simulink model "v3"  (R2023a)
settings: Solver=VariableStepAuto  StartTime=0.0  StopTime=4  RelTol=1e-3
libraries: dspvision x9, simulink x7, commsrccod2 x6, dspsigops x4, dspfdesign x4, commfilt2 x3, commchan3 x1, commsink2 x1
settings Model: Creator=zizim  LastModifiedBy=zizim
settings OptimizationCC: BlockReduction=off  ConditionallyExecuteInputs=off

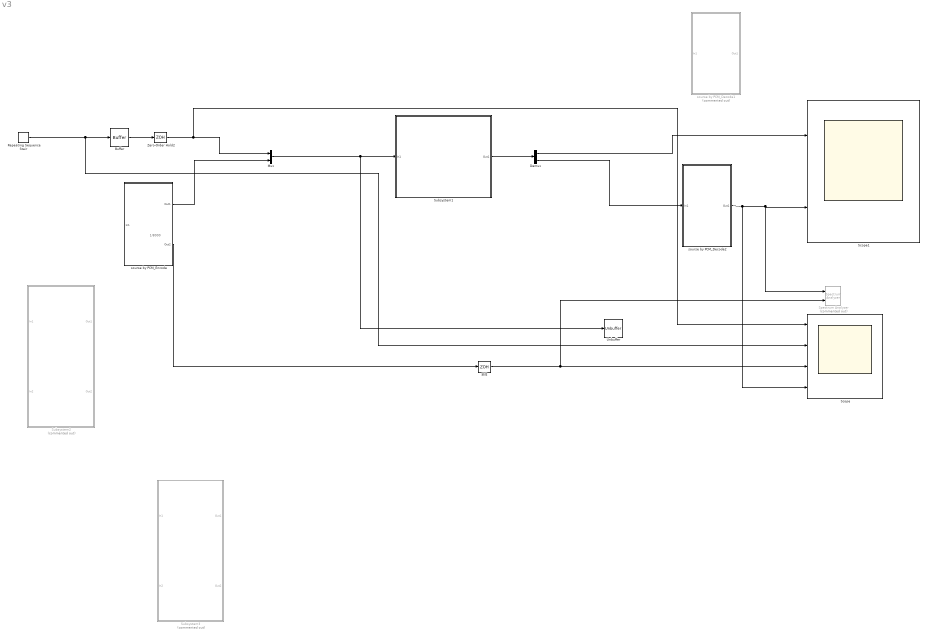
== system v3 ==
  note: 1/8000
  Buffer : Buffer  N=8  OutputFrames=off
  Demux : Demux  Outputs=2
  Mux : Mux  Inputs=2
  Repeating Sequence Stair : simulink/Sources/Repeating Sequence Stair  OutValues=[1 1 0 0 0 1 1 1]  tsamp=1/8000  OutMin=[]  OutMax=[]  OutDataTypeStr=double  OutputDataTypeScalingMode=double  OutDataType=fixdt(0,8)  ConRadixGroup=Best Precision: Vector-wise  OutScaling=2^-12
  Scope : Scope  NumInputPorts=4
  Scope1 : Scope  NumInputPorts=2
  Spectrum Analyzer : SpectrumAnalyzer  Commented=on  NumInputPorts=2  WindowPosition=[323.000000,237.000000,718.000000,504.000000,]  ScopeFrameLocation=window  Span=8000  StartFrequency=-4000  StopFrequency=4000  YLimits=[-105.37237061,9.4990938]  ColorLimits=[-80 20]  ShowLegend=on
  Subsystem1 : Subsystem
  Subsystem2 : Subsystem  Commented=on
  Subsystem3 : Subsystem  Commented=on
  Unbuffer : Unbuffer
  Zero-Order Hold2 : ZeroOrderHold  SampleTime=1/8000
  sourse by PCM_Decode1 : Subsystem  Commented=on
  sourse by PCM_Decode2 : Subsystem
  sourse by PCM_Encode : Subsystem
  采样 : ZeroOrderHold  SampleTime=1/64000
  wires:
  sourse by PCM_Encode/2(Out2) -> 采样/1
  采样/1 -> Spectrum Analyzer/2, Scope/3
  Mux/1 -> Unbuffer/1, Subsystem1/1(In1)
  sourse by PCM_Decode2/1(Out1) -> Scope/4, Spectrum Analyzer/1, Scope1/2
  Repeating Sequence Stair/1 -> Scope/2, Buffer/1
  Buffer/1 -> Zero-Order Hold2/1
  Zero-Order Hold2/1 -> Scope/1, Mux/1
  sourse by PCM_Encode/1(Out1) -> Mux/2
  Subsystem1/1(Out1) -> Demux/1
  Demux/2 -> sourse by PCM_Decode2/1(In1)
  Demux/1 -> Scope1/1

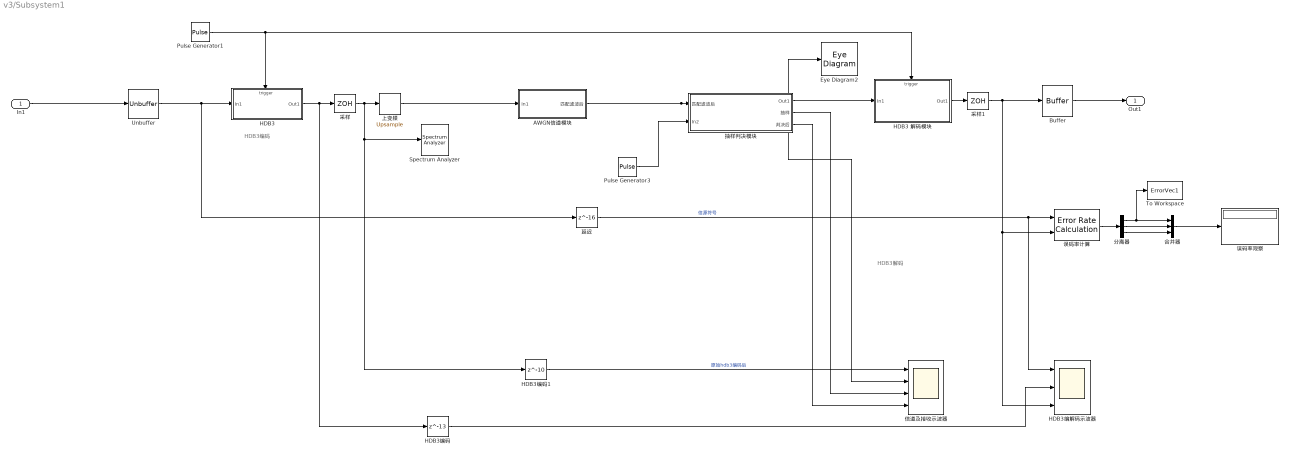
== system v3/Subsystem1 ==
  note: HDB3解码
  note: HDB3编码
  In1 : Inport
  AWGN信道模块 : Subsystem
  Buffer : Buffer  N=16  OutputFrames=off
  Eye Diagram2 : EyeDiagram
  HDB3 : Subsystem  TreatAsAtomicUnit=on
  HDB3 解码模块 : Subsystem  Tag=decode  Description=decode1  TreatAsAtomicUnit=on
  HDB3编码 : Delay  DelayLength=13  InitialCondition=0  SampleTime=1/128000
  HDB3编码1 : Delay  DelayLength=10  InitialCondition=0  SampleTime=1/128000
  HDB3编解码示波器 : Scope  NumInputPorts=3
  Pulse Generator1 : DiscretePulseGenerator  Period=10  PulseWidth=5  SampleTime=1/1280000
  Pulse Generator3 : DiscretePulseGenerator  Period=10  PulseWidth=5  SampleTime=1/1280000
  Spectrum Analyzer : SpectrumAnalyzer  WindowPosition=[507.000000,152.000000,800.000000,451.000000,]  ScopeFrameLocation=window  Method=Welch  SampleRate=1000  AxesScaling=Manual  Span=1000  StartFrequency=-500  StopFrequency=500  AveragingMethod=Running  YLimits=[-78.858739814638965981,15.222011316412805471]
      settings: OpenAtSimulationStart=off
  To Workspace : ToWorkspace  VariableName=ErrorVec1  SampleTime=-1
      settings: Save2DSignal=2-D array (concatenate along first dimension)
  Unbuffer : Unbuffer
  上变频 : dspsigops/Upsample  FactorSource=Dialog parameter  N=10  Nmax=16  phase=0  InputProcessing=Columns as channels (frame based)  RateOptions=Allow multirate processing  ic=0  mode=Unused parameter value
  信道及接收示波器 : Scope  NumInputPorts=4
  分离器 : Demux  Outputs=3
  合并器 : Mux  Inputs=3
  延迟 : Delay  DelayLength=16  InitialCondition=0  SampleTime=1/128000
  抽样判决模块 : Subsystem
  误码率观察 : Display
  误码率计算 : commsink2/Error Rate Calculation  N=0  st_delay=0  cp_mode=Entire frame  subframe=[]  PMode=Port  WsName=ErrorVec  RsMode2=off  stop=off  numErr=100  maxBits=1e6
  采样 : ZeroOrderHold  SampleTime=1/128000
  采样1 : ZeroOrderHold  SampleTime=1/128000
  Out1 : Outport
  wires:
  HDB3 解码模块/1(Out1) -> 采样1/1
  AWGN信道模块/1(匹配滤波后) -> 信道及接收示波器/2, Eye Diagram2/1, 抽样判决模块/1(匹配滤波后)
  分离器/2 -> 合并器/2
  采样/1 -> HDB3编码1/1, Spectrum Analyzer/1, 上变频/1
  HDB3/1(Out1) -> HDB3编码/1, 采样/1
  Pulse Generator1/1 -> HDB3 解码模块/Trigger, HDB3/Trigger
  分离器/3 -> 合并器/3
  上变频/1 -> AWGN信道模块/1(In1)
  抽样判决模块/2(抽样) -> 信道及接收示波器/3
  延迟/1 -> HDB3编解码示波器/1, 误码率计算/1  "信源符号"
  分离器/1 -> To Workspace/1, 合并器/1
  HDB3编码1/1 -> 信道及接收示波器/1  "原始hdb3编码后"
  合并器/1 -> 误码率观察/1
  Pulse Generator3/1 -> 抽样判决模块/2(In2)
  误码率计算/1 -> 分离器/1
  抽样判决模块/3(判决后) -> 信道及接收示波器/4
  HDB3编码/1 -> HDB3编解码示波器/2
  抽样判决模块/1(Out1) -> HDB3 解码模块/1(In1)
  采样1/1 -> Buffer/1, 误码率计算/2, HDB3编解码示波器/3
  In1/1 -> Unbuffer/1
  Unbuffer/1 -> 延迟/1, HDB3/1(In1)
  Buffer/1 -> Out1/1

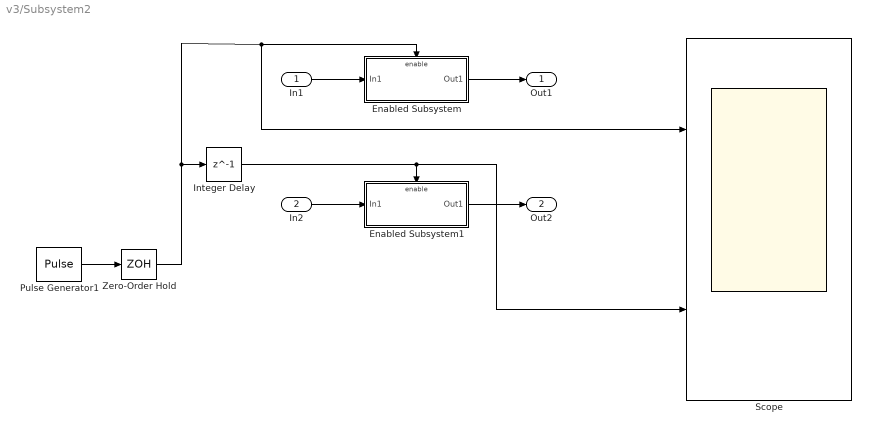
== system v3/Subsystem2 ==
  In1 : Inport
  In2 : Inport  Port=2
  Enabled Subsystem : Subsystem  TreatAsAtomicUnit=on
  Enabled Subsystem1 : Subsystem  TreatAsAtomicUnit=on
  Integer Delay : Delay  DelayLength=1
  Pulse Generator1 : DiscretePulseGenerator  PulseType=Time based  Amplitude=3  Period=1/160000  PulseWidth=1/320000  SampleTime=1/640000
  Scope : Scope  NumInputPorts=2
  Zero-Order Hold : ZeroOrderHold  SampleTime=1/320000
  Out1 : Outport
  Out2 : Outport  Port=2
  wires:
  Zero-Order Hold/1 -> Scope/1, Enabled Subsystem/Enable, Integer Delay/1
  Integer Delay/1 -> Scope/2, Enabled Subsystem1/Enable
  Pulse Generator1/1 -> Zero-Order Hold/1
  Enabled Subsystem/1(Out1) -> Out1/1
  In1/1 -> Enabled Subsystem/1(In1)
  In2/1 -> Enabled Subsystem1/1(In1)
  Enabled Subsystem1/1(Out1) -> Out2/1

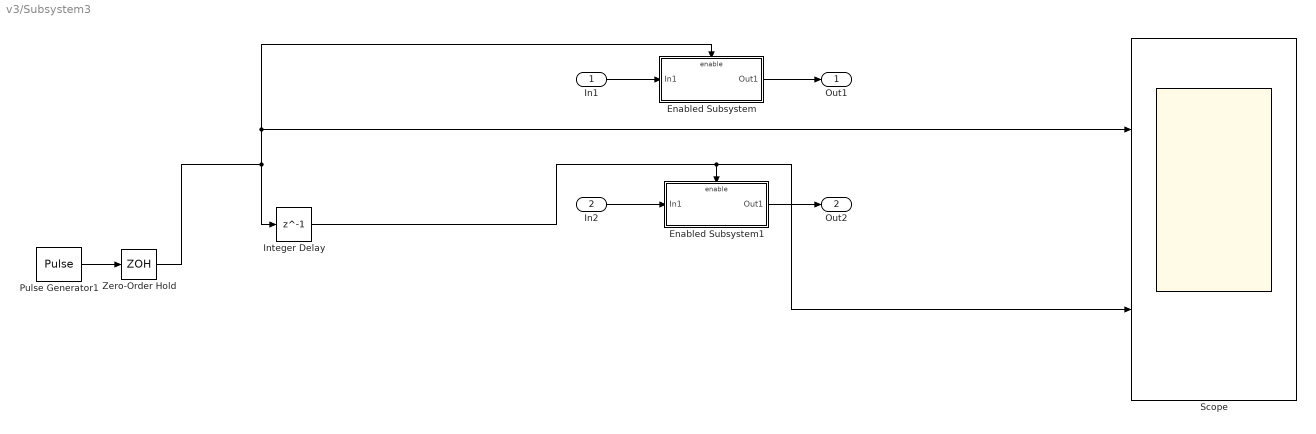
== system v3/Subsystem3 ==
  In1 : Inport
  In2 : Inport  Port=2
  Enabled Subsystem : Subsystem  TreatAsAtomicUnit=on
  Enabled Subsystem1 : Subsystem  TreatAsAtomicUnit=on
  Integer Delay : Delay  DelayLength=1
  Pulse Generator1 : DiscretePulseGenerator  PulseType=Time based  Amplitude=3  Period=1/160000  PulseWidth=1/320000  SampleTime=1/640000
  Scope : Scope  NumInputPorts=2
  Zero-Order Hold : ZeroOrderHold  SampleTime=1/32000
  Out1 : Outport
  Out2 : Outport  Port=2
  wires:
  Zero-Order Hold/1 -> Enabled Subsystem/Enable, Scope/1, Integer Delay/1
  Pulse Generator1/1 -> Zero-Order Hold/1
  Enabled Subsystem/1(Out1) -> Out1/1
  In1/1 -> Enabled Subsystem/1(In1)
  In2/1 -> Enabled Subsystem1/1(In1)
  Enabled Subsystem1/1(Out1) -> Out2/1
  Integer Delay/1 -> Scope/2, Enabled Subsystem1/Enable

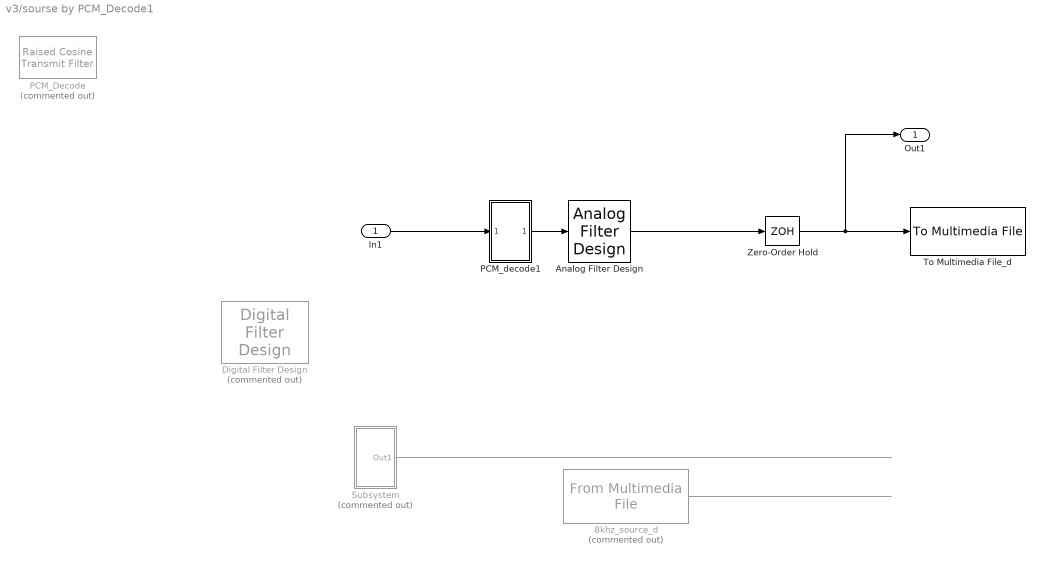
== system v3/sourse by PCM_Decode1 ==
  In1 : Inport
  8khz_source_d : dspvision/From Multimedia File  Commented=on  inputFilename=E:\Matlab\toolbox\dsp\samples\speech_dft_8kHz.wav  readRange=[1 Inf]  loop=on  numPlays=inf  outputStreams=Audio only  videoDataType=single  audioDataType=double  inheritSampleTime=on  userDefinedSampleTime=1/30  noAudioOutput=off  isIntensityVideo=off  fourcc=RGB  colorVideoFormat=Separate color signals  outputEOF=off  dataOrg=Column-major  audioFrameSize=1  computeAudioFrameSize=off  outSamplingMode=Sample based
      settings: LibrarySourceBlock=audiosources/From Multimedia File
  Analog Filter Design : dspfdesign/Analog Filter Design  method=Chebyshev II  filttype=Lowpass  N=8  Wlo=2*pi*3400  Whi=80  Rp=2  Rs=40
  Digital Filter Design : dspfdesign/Digital Filter Design  Commented=on  mwdsp_browser_bugfix_var=off
  PCM_Decode : commfilt2/Raised Cosine Transmit Filter  Commented=on  filtType=Square root  R=0.  filtSpan=10  N=8  filterGain=1  RateOptions=Allow multirate processing  framing=Mute  checkCoeff=off  variableName=rcTxFilt1  checkGain=Normalized  sampMode=Mute  saveAsFlag=0  currentFiltSpan=10  D=5  launchFVT=on  roundingMode=Floor  overflowMode=off  coeffDataTypeStr=Inherit: Same word length as input  coeffMin=[]  coeffMax=[]  coeffLastDataTypeStr=Inherit: Same word length as input  outputMin=[]  outputMax=[]
      settings: LibrarySourceBlock=|
      | commhdlfilt/Raised Cosine
      | Transmit Filter
  PCM_decode1 : Subsystem
  Subsystem : Subsystem  Commented=on
  To Multimedia File_d : dspvision/To Multimedia File  outputFilename=G:\zizim\Documents\code\Matlab\combine_system_hdb3\PCM_Decode_d.wav  streamSelection=Audio only  videoCompressor=None (uncompressed)  audioCompressor=None (uncompressed)  imagePorts=Separate color signals  fileType=WAV  audioDatatype=16-bit integer  fourcc=RGB  videoQuality=75  mj2000CompFactor=10
      settings: LibrarySourceBlock=audiosinks/To Multimedia File
  Zero-Order Hold : ZeroOrderHold  SampleTime=1/8000
  Out1 : Outport
  wires:
  Zero-Order Hold/1 -> Out1/1, To Multimedia File_d/1
  8khz_source_d/1 -> ?
  In1/1 -> PCM_decode1/1(In1)
  PCM_decode1/1(Out1) -> Analog Filter Design/1
  Subsystem/1(Out1) -> ?
  Analog Filter Design/1 -> Zero-Order Hold/1

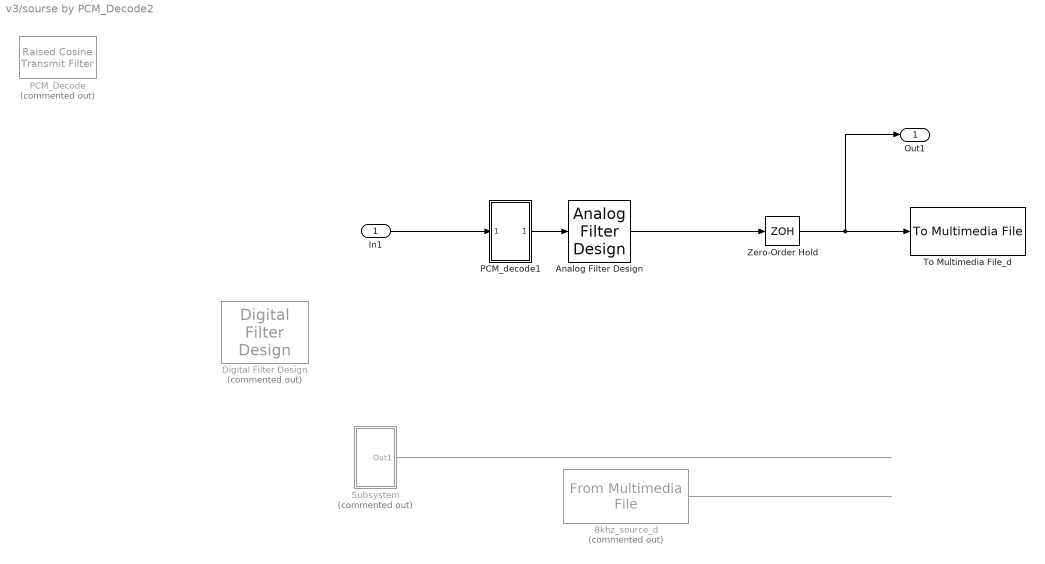
== system v3/sourse by PCM_Decode2 ==
  In1 : Inport
  8khz_source_d : dspvision/From Multimedia File  Commented=on  inputFilename=E:\Matlab\toolbox\dsp\samples\speech_dft_8kHz.wav  readRange=[1 Inf]  loop=on  numPlays=inf  outputStreams=Audio only  videoDataType=single  audioDataType=double  inheritSampleTime=on  userDefinedSampleTime=1/30  noAudioOutput=off  isIntensityVideo=off  fourcc=RGB  colorVideoFormat=Separate color signals  outputEOF=off  dataOrg=Column-major  audioFrameSize=1  computeAudioFrameSize=off  outSamplingMode=Sample based
      settings: LibrarySourceBlock=audiosources/From Multimedia File
  Analog Filter Design : dspfdesign/Analog Filter Design  method=Chebyshev II  filttype=Lowpass  N=8  Wlo=2*pi*3400  Whi=80  Rp=2  Rs=40
  Digital Filter Design : dspfdesign/Digital Filter Design  Commented=on  mwdsp_browser_bugfix_var=off
  PCM_Decode : commfilt2/Raised Cosine Transmit Filter  Commented=on  filtType=Square root  R=0.  filtSpan=10  N=8  filterGain=1  RateOptions=Allow multirate processing  framing=Mute  checkCoeff=off  variableName=rcTxFilt1  checkGain=Normalized  sampMode=Mute  saveAsFlag=0  currentFiltSpan=10  D=5  launchFVT=on  roundingMode=Floor  overflowMode=off  coeffDataTypeStr=Inherit: Same word length as input  coeffMin=[]  coeffMax=[]  coeffLastDataTypeStr=Inherit: Same word length as input  outputMin=[]  outputMax=[]
      settings: LibrarySourceBlock=|
      | commhdlfilt/Raised Cosine
      | Transmit Filter
  PCM_decode1 : Subsystem
  Subsystem : Subsystem  Commented=on
  To Multimedia File_d : dspvision/To Multimedia File  outputFilename=G:\zizim\Documents\UJN_HomeWork\通信原理仿真\communication_project\temp\PCM_Decode_d.wav  streamSelection=Audio only  videoCompressor=None (uncompressed)  audioCompressor=None (uncompressed)  imagePorts=Separate color signals  fileType=WAV  audioDatatype=16-bit integer  fourcc=RGB  videoQuality=75  mj2000CompFactor=10
      settings: LibrarySourceBlock=audiosinks/To Multimedia File
  Zero-Order Hold : ZeroOrderHold  SampleTime=1/8000
  Out1 : Outport
  wires:
  Zero-Order Hold/1 -> Out1/1, To Multimedia File_d/1
  8khz_source_d/1 -> ?
  In1/1 -> PCM_decode1/1(In1)
  PCM_decode1/1(Out1) -> Analog Filter Design/1
  Subsystem/1(Out1) -> ?
  Analog Filter Design/1 -> Zero-Order Hold/1

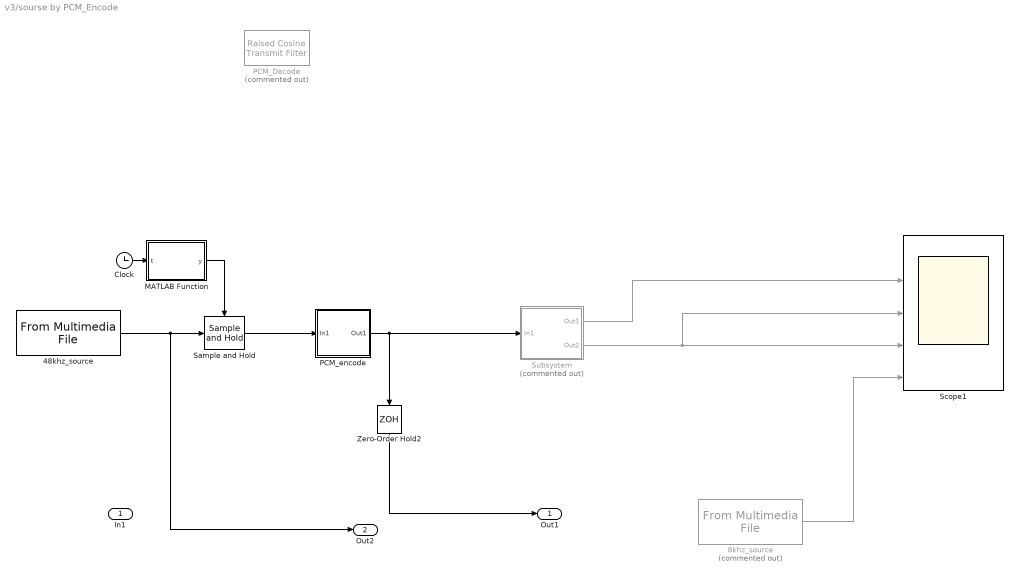
== system v3/sourse by PCM_Encode ==
  In1 : Inport
  48khz_source : dspvision/From Multimedia File  inputFilename=E:\Matlab\toolbox\dsp\samples\speech_dft_8kHz.wav  readRange=[1 Inf]  loop=on  numPlays=inf  outputStreams=Audio only  videoDataType=single  audioDataType=double  inheritSampleTime=on  userDefinedSampleTime=1/30  noAudioOutput=off  isIntensityVideo=off  fourcc=RGB  colorVideoFormat=Separate color signals  outputEOF=off  dataOrg=Column-major  audioFrameSize=1  computeAudioFrameSize=off  outSamplingMode=Sample based
      settings: LibrarySourceBlock=audiosources/From Multimedia File
  8khz_source : dspvision/From Multimedia File  Commented=on  inputFilename=E:\Matlab\toolbox\dsp\samples\speech_dft_8kHz.wav  readRange=[1 Inf]  loop=on  numPlays=inf  outputStreams=Audio only  videoDataType=single  audioDataType=double  inheritSampleTime=on  userDefinedSampleTime=1/30  noAudioOutput=off  isIntensityVideo=off  fourcc=RGB  colorVideoFormat=Separate color signals  outputEOF=off  dataOrg=Column-major  audioFrameSize=1  computeAudioFrameSize=off  outSamplingMode=Sample based
      settings: LibrarySourceBlock=audiosources/From Multimedia File
  Clock : Clock
      settings: Decimation=4
  MATLAB Function : MATLAB Function  TreatAsAtomicUnit=on
  PCM_Decode : commfilt2/Raised Cosine Transmit Filter  Commented=on  filtType=Square root  R=0.  filtSpan=10  N=8  filterGain=1  RateOptions=Allow multirate processing  framing=Mute  checkCoeff=off  variableName=rcTxFilt1  checkGain=Normalized  sampMode=Mute  saveAsFlag=0  currentFiltSpan=10  D=5  launchFVT=on  roundingMode=Floor  overflowMode=off  coeffDataTypeStr=Inherit: Same word length as input  coeffMin=[]  coeffMax=[]  coeffLastDataTypeStr=Inherit: Same word length as input  outputMin=[]  outputMax=[]
      settings: LibrarySourceBlock=|
      | commhdlfilt/Raised Cosine
      | Transmit Filter
  PCM_encode : Subsystem
  Sample and Hold : dspsigops/Sample and Hold  trig=Rising edge  initCond=0  latchinput=off
  Scope1 : Scope  NumInputPorts=5
  Subsystem : Subsystem  Commented=on
  Zero-Order Hold2 : ZeroOrderHold  SampleTime=1/8000
  Out1 : Outport
  Out2 : Outport  Port=2
  wires:
  8khz_source/1 -> Scope1/5
  Clock/1 -> MATLAB Function/1(t)
  MATLAB Function/1(y) -> Sample and Hold/Trigger
  Sample and Hold/1 -> PCM_encode/1(In1)
  Subsystem/2(Out2) -> Scope1/3, Scope1/4
  Subsystem/1(Out1) -> Scope1/2
  48khz_source/1 -> Out2/1, Sample and Hold/1
  PCM_encode/1(Out1) -> Zero-Order Hold2/1, Subsystem/1(In1)
  Zero-Order Hold2/1 -> Out1/1

== system v3/Subsystem1/AWGN信道模块 ==
  note: 信道模块
  In1 : Inport
  信道 : commchan3/AWGN Channel  LegacyMode=on  NoiseMethod="Signal to noise ratio  (SNR)"  noiseMode="Signal to noise ratio  (SNR)"  EbNo=10  EsNo=10  SNR=10000  BitsPerSymbol=1  SignalPower=1  SamplesPerSymbol=1  SymbolPeriod=1  VarianceSource=Parameter  Variance=1  RandomStream=Global stream  Seed=67  SimulateUsing=Code generation
  匹配滤波器 : DiscreteFilter  Numerator=[ rcosdesign(0.2,10,10,'sqrt')]  Denominator=[1]  SampleTime=1/1280000
  发射滤波器 : DiscreteFilter  Numerator=[ rcosdesign(0.2,10,10,'sqrt')]  Denominator=[1]  SampleTime=1/1280000
  匹配滤波后 : Outport
  wires:
  匹配滤波器/1 -> 匹配滤波后/1  "匹配滤波后"
  信道/1 -> 匹配滤波器/1
  In1/1 -> 发射滤波器/1
  发射滤波器/1 -> 信道/1

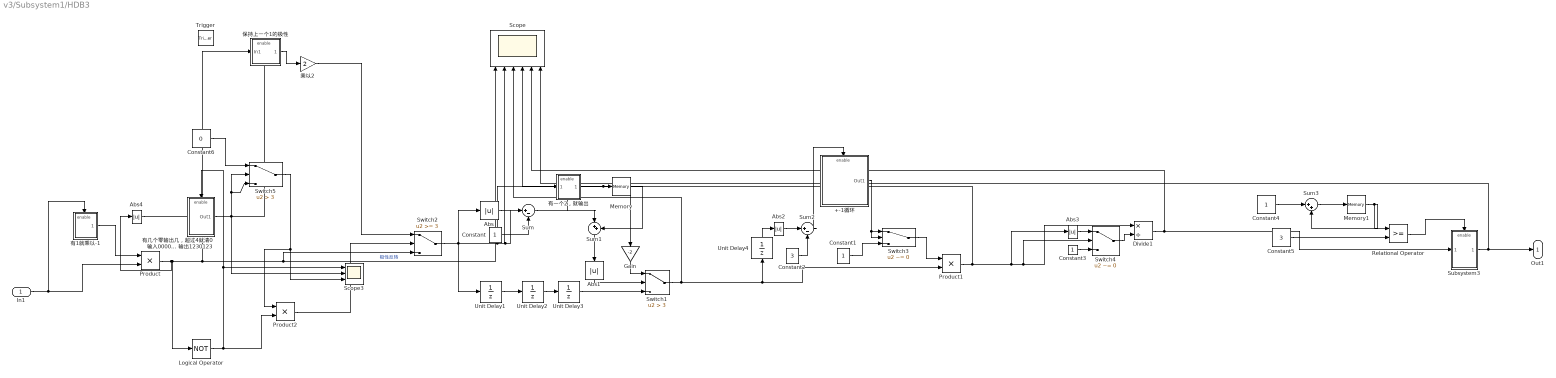
== system v3/Subsystem1/HDB3 ==
  In1 : Inport
  Trigger : TriggerPort  VariantControl=Variant
  +-1循环 : Subsystem
  Abs{,1..4} (5 alike) : Abs  SaturateOnIntegerOverflow=off
  Constant{,1,3..4} (4 alike) : Constant
  Constant2 : Constant  Value=3
  Constant5 : Constant  Value=3
  Constant6 : Constant  Value=0
  Divide1 : Product  Inputs=*/
  Gain : Gain  Gain=-2
  Logical Operator : Logic  Operator=NOT  AllPortsSameDT=off  OutDataTypeStr=boolean
  Memory : Memory  InheritSampleTime=on
  Memory1 : Memory  InheritSampleTime=on
  Product : Product  RndMeth=Zero
  Product1 : Product  RndMeth=Zero
  Product2 : Product  RndMeth=Zero
  Relational Operator : RelationalOperator  OutDataTypeStr=boolean  InputSameDT=off
  Scope : Scope  NumInputPorts=6
  Scope3 : Scope  NumInputPorts=3
  Subsystem3 : Subsystem
  Sum : Sum  Inputs=|+-
  Sum1 : Sum  Inputs=|++
  Sum2 : Sum  Inputs=|+-
  Sum3 : Sum  Inputs=|++
  Switch1 : Switch  Criteria=u2 > Threshold  Threshold=3  SaturateOnIntegerOverflow=off  InputSameDT=off
  Switch2 : Switch  Threshold=3  SaturateOnIntegerOverflow=off  InputSameDT=off
  Switch3 : Switch  Criteria=u2 ~= 0  Threshold=3  SaturateOnIntegerOverflow=off  InputSameDT=off
  Switch4 : Switch  Criteria=u2 ~= 0  Threshold=3  SaturateOnIntegerOverflow=off  InputSameDT=off
  Switch5 : Switch  Criteria=u2 > Threshold  Threshold=3  SaturateOnIntegerOverflow=off  InputSameDT=off
  Unit Delay{1..4} (4 alike) : UnitDelay  SampleTime=-1  HasFrameUpgradeWarning=on
  乘以2 : Gain  Gain=2
  保持上一个1的极性 : Subsystem
  有1就乘以-1 : Subsystem
  有一个2，就输出 : Subsystem
  有几个零输出几，超过4就清0 输入0000000 输出1230123 : Subsystem
  Out1 : Outport
  wires:
  In1/1 -> 有1就乘以-1/Enable, Product/2
  Memory1/1 -> Sum3/2, Relational Operator/1
  Subsystem3/1(Out1) -> Out1/1, Scope/6
  Constant5/1 -> Relational Operator/2
  Relational Operator/1 -> Subsystem3/Enable
  Divide1/1 -> Scope/5, Subsystem3/1(In2)
  Constant4/1 -> Sum3/1
  Sum3/1 -> Memory1/1
  Sum1/1 -> Abs1/1
  Abs1/1 -> Switch1/2
  Abs/1 -> Sum/1
  Sum2/1 -> +-1循环/Enable
  Constant/1 -> Sum/2
  Sum/1 -> 有一个2，就输出/Enable
  +-1循环/1(Out1) -> Switch3/2, Switch3/1
  有一个2，就输出/1(Out1) -> Gain/1, Memory/1
  Memory/1 -> Sum1/2
  Unit Delay3/1 -> Switch1/3
  Gain/1 -> Switch1/1
  Unit Delay1/1 -> Unit Delay2/1
  Switch3/1 -> Product1/1
  Switch4/1 -> Divide1/2
  Constant2/1 -> Sum2/2
  Switch1/1 -> Product1/2, Unit Delay4/1, Scope/3
  Unit Delay4/1 -> Abs2/1
  Abs3/1 -> Switch4/1
  Abs2/1 -> Sum2/1
  Constant3/1 -> Switch4/3
  Constant1/1 -> Switch3/3
  乘以2/1 -> Switch2/1
  Product1/1 -> Switch4/2, Divide1/1, Abs3/1, Scope/4
  有1就乘以-1/1(Out1) -> Product/1
  Product/1 -> Switch2/3, Scope/1, 保持上一个1的极性/1(In1), Logical Operator/1, Abs4/1  "极性反转"
  Unit Delay2/1 -> Unit Delay3/1
  Switch2/1 -> Sum1/1, Scope/2, 有一个2，就输出/1(In1), Abs/1, Unit Delay1/1
  保持上一个1的极性/1(Out1) -> 乘以2/1
  Product2/1 -> Switch2/2
  Abs4/1 -> 保持上一个1的极性/Enable
  有几个零输出几，超过4就清0 输入0000000 输出1230123/1(Out1) -> Switch5/3, Switch5/2, Scope3/2
  Constant6/1 -> Switch5/1
  Logical Operator/1 -> Product2/2, 有几个零输出几，超过4就清0 输入0000000 输出1230123/Enable, Scope3/1
  Switch5/1 -> Product2/1, Scope3/3

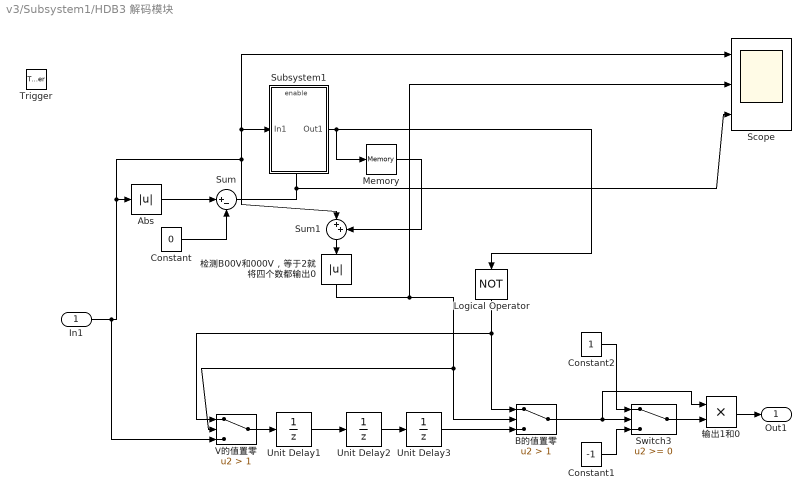
== system v3/Subsystem1/HDB3 解码模块 ==
  In1 : Inport
  Trigger : TriggerPort  VariantControl=Variant
  Abs : Abs  SaturateOnIntegerOverflow=off
  B的值置零 : Switch  Criteria=u2 > Threshold  Threshold=1  SaturateOnIntegerOverflow=off  InputSameDT=off
  Constant : Constant  Value=0
  Constant1 : Constant  Value=-1
  Constant2 : Constant
  Logical Operator : Logic  Operator=NOT  AllPortsSameDT=off  OutDataTypeStr=boolean
  Memory : Memory  InheritSampleTime=on
  Scope : Scope  NumInputPorts=3
  Subsystem1 : Subsystem
  Sum : Sum  Inputs=|+-
  Sum1 : Sum  Inputs=|++
  Switch3 : Switch  SaturateOnIntegerOverflow=off  InputSameDT=off
  Unit Delay1 : UnitDelay  SampleTime=-1  HasFrameUpgradeWarning=on
  Unit Delay2 : UnitDelay  SampleTime=-1  HasFrameUpgradeWarning=on
  Unit Delay3 : UnitDelay  SampleTime=-1  HasFrameUpgradeWarning=on
  V的值置零 : Switch  Criteria=u2 > Threshold  Threshold=1  SaturateOnIntegerOverflow=off  InputSameDT=off
  检测B00V和000V，等于2就将四个数都输出0 : Abs  SaturateOnIntegerOverflow=off
  输出1和0 : Product  RndMeth=Zero
  Out1 : Outport
  wires:
  In1/1 -> V的值置零/3, Subsystem1/1(In1), Scope/1, Sum1/1, Abs/1
  Constant/1 -> Sum/2
  Abs/1 -> Sum/1
  Sum/1 -> Scope/3, Subsystem1/Enable
  Subsystem1/1(Out1) -> Memory/1, Logical Operator/1
  Memory/1 -> Sum1/2
  Sum1/1 -> 检测B00V和000V，等于2就将四个数都输出0/1
  检测B00V和000V，等于2就将四个数都输出0/1 -> Scope/2, B的值置零/2, V的值置零/2
  Logical Operator/1 -> V的值置零/1, B的值置零/1
  Unit Delay3/1 -> B的值置零/3
  Unit Delay1/1 -> Unit Delay2/1
  Unit Delay2/1 -> Unit Delay3/1
  V的值置零/1 -> Unit Delay1/1
  B的值置零/1 -> Switch3/2, 输出1和0/1
  Constant1/1 -> Switch3/3
  Constant2/1 -> Switch3/1
  Switch3/1 -> 输出1和0/2
  输出1和0/1 -> Out1/1

== system v3/Subsystem1/抽样判决模块 ==
  匹配滤波后 : Inport
  In2 : Inport  Port=2
  Downsample1 : DownSample  N=10  InputProcessing=Inherited (this choice will be removed - see release notes)  RateOptions=Allow multirate processing
  判决 : Subsystem
  每隔抽样 : Subsystem  TreatAsAtomicUnit=on
  Out1 : Outport
  抽样 : Outport  Port=2
  判决后 : Outport  Port=3
  wires:
  Downsample1/1 -> Out1/1
  匹配滤波后/1 -> 每隔抽样/1(In1)
  判决/1(Out1) -> 判决后/1, Downsample1/1  "判决后"
  每隔抽样/1(Out1) -> 抽样/1, 判决/1(In1)  "抽样"
  In2/1 -> 每隔抽样/Trigger

== system v3/Subsystem2/Enabled Subsystem ==
  In1 : Inport
  Enable : EnablePort
  Out1 : Outport
  wires:
  In1/1 -> Out1/1

== system v3/Subsystem2/Enabled Subsystem1 ==
  In1 : Inport
  Enable : EnablePort
  Out1 : Outport
  wires:
  In1/1 -> Out1/1

== system v3/Subsystem3/Enabled Subsystem ==
  In1 : Inport
  Enable : EnablePort
  Out1 : Outport
  wires:
  In1/1 -> Out1/1

== system v3/Subsystem3/Enabled Subsystem1 ==
  In1 : Inport
  Enable : EnablePort
  Out1 : Outport
  wires:
  In1/1 -> Out1/1

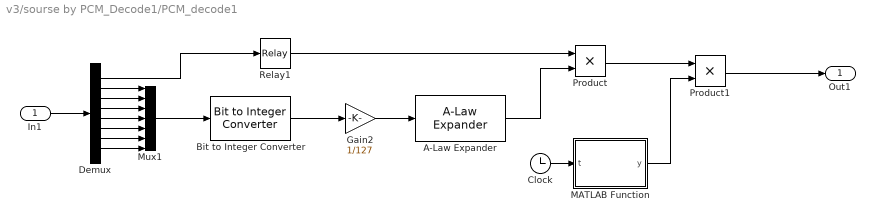
== system v3/sourse by PCM_Decode1/PCM_decode1 ==
  In1 : Inport
  A-Law Expander : commsrccod2/A-Law Expander  A=87.6  V=1
  Bit to Integer Converter : simulink/Logic and Bit Operations/Bit to Integer Converter  nbits=7  bitOrder=MSB first  signedOutputValues=Unsigned  outDtype=double  outDtypeSigned=Inherit via internal rule
      settings: LibrarySourceBlock=|
      | commutil2/Bit to Integer
      | Converter
  Clock : Clock
      settings: Decimation=4
  Demux : Demux  Outputs=8
  Gain2 : Gain  Gain=1/127
  MATLAB Function : MATLAB Function  TreatAsAtomicUnit=on
  Mux1 : Mux  Inputs=7
  Product : Product
  Product1 : Product
  Relay1 : Relay  OnSwitchValue=0.9  OffOutputValue=-1
  Out1 : Outport
  wires:
  In1/1 -> Demux/1
  Relay1/1 -> Product/1
  Demux/5 -> Mux1/4
  Mux1/1 -> Bit to Integer Converter/1
  Demux/1 -> Relay1/1
  Demux/4 -> Mux1/3
  Gain2/1 -> A-Law Expander/1
  Demux/6 -> Mux1/5
  Demux/7 -> Mux1/6
  Bit to Integer Converter/1 -> Gain2/1
  Demux/2 -> Mux1/1
  Demux/3 -> Mux1/2
  A-Law Expander/1 -> Product/2
  Demux/8 -> Mux1/7
  Product/1 -> Product1/1
  Product1/1 -> Out1/1
  MATLAB Function/1(y) -> Product1/2
  Clock/1 -> MATLAB Function/1(t)

== system v3/sourse by PCM_Decode1/Subsystem ==
  48khz_source_d : dspvision/From Multimedia File  inputFilename=E:\Matlab\toolbox\dsp\samples\audio48kHz.wav  readRange=[1 Inf]  loop=on  numPlays=inf  outputStreams=Audio only  videoDataType=single  audioDataType=double  inheritSampleTime=on  userDefinedSampleTime=1/30  noAudioOutput=off  isIntensityVideo=off  fourcc=RGB  colorVideoFormat=Separate color signals  outputEOF=off  dataOrg=Column-major  audioFrameSize=1  computeAudioFrameSize=off  outSamplingMode=Sample based
      settings: LibrarySourceBlock=audiosources/From Multimedia File
  Clock : Clock
      settings: Decimation=4
  MATLAB Function : MATLAB Function  TreatAsAtomicUnit=on
  PCM_encode_d : Subsystem
  Sample and Hold : dspsigops/Sample and Hold  trig=Rising edge  initCond=0  latchinput=off
  Out1 : Outport
  wires:
  Clock/1 -> MATLAB Function/1(t)
  Sample and Hold/1 -> PCM_encode_d/1(In1)
  48khz_source_d/1 -> Sample and Hold/1
  MATLAB Function/1(y) -> Sample and Hold/Trigger
  PCM_encode_d/1(Out1) -> Out1/1

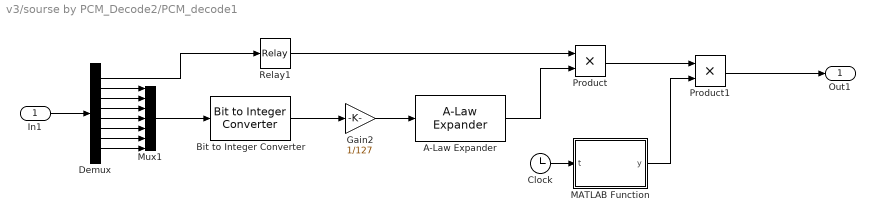
== system v3/sourse by PCM_Decode2/PCM_decode1 ==
  In1 : Inport
  A-Law Expander : commsrccod2/A-Law Expander  A=87.6  V=1
  Bit to Integer Converter : simulink/Logic and Bit Operations/Bit to Integer Converter  nbits=7  bitOrder=MSB first  signedOutputValues=Unsigned  outDtype=double  outDtypeSigned=Inherit via internal rule
      settings: LibrarySourceBlock=|
      | commutil2/Bit to Integer
      | Converter
  Clock : Clock
      settings: Decimation=4
  Demux : Demux  Outputs=8
  Gain2 : Gain  Gain=1/127
  MATLAB Function : MATLAB Function  TreatAsAtomicUnit=on
  Mux1 : Mux  Inputs=7
  Product : Product
  Product1 : Product
  Relay1 : Relay  OnSwitchValue=0.9  OffOutputValue=-1
  Out1 : Outport
  wires:
  In1/1 -> Demux/1
  Relay1/1 -> Product/1
  Demux/5 -> Mux1/4
  Mux1/1 -> Bit to Integer Converter/1
  Demux/1 -> Relay1/1
  Demux/4 -> Mux1/3
  Gain2/1 -> A-Law Expander/1
  Demux/6 -> Mux1/5
  Demux/7 -> Mux1/6
  Bit to Integer Converter/1 -> Gain2/1
  Demux/2 -> Mux1/1
  Demux/3 -> Mux1/2
  A-Law Expander/1 -> Product/2
  Demux/8 -> Mux1/7
  Product/1 -> Product1/1
  Product1/1 -> Out1/1
  MATLAB Function/1(y) -> Product1/2
  Clock/1 -> MATLAB Function/1(t)

== system v3/sourse by PCM_Decode2/Subsystem ==
  48khz_source_d : dspvision/From Multimedia File  inputFilename=E:\Matlab\toolbox\dsp\samples\audio48kHz.wav  readRange=[1 Inf]  loop=on  numPlays=inf  outputStreams=Audio only  videoDataType=single  audioDataType=double  inheritSampleTime=on  userDefinedSampleTime=1/30  noAudioOutput=off  isIntensityVideo=off  fourcc=RGB  colorVideoFormat=Separate color signals  outputEOF=off  dataOrg=Column-major  audioFrameSize=1  computeAudioFrameSize=off  outSamplingMode=Sample based
      settings: LibrarySourceBlock=audiosources/From Multimedia File
  Clock : Clock
      settings: Decimation=4
  MATLAB Function : MATLAB Function  TreatAsAtomicUnit=on
  PCM_encode_d : Subsystem
  Sample and Hold : dspsigops/Sample and Hold  trig=Rising edge  initCond=0  latchinput=off
  Out1 : Outport
  wires:
  Clock/1 -> MATLAB Function/1(t)
  Sample and Hold/1 -> PCM_encode_d/1(In1)
  48khz_source_d/1 -> Sample and Hold/1
  MATLAB Function/1(y) -> Sample and Hold/Trigger
  PCM_encode_d/1(Out1) -> Out1/1

== system v3/sourse by PCM_Encode/PCM_encode ==
  In1 : Inport
  A-Law Compressor : commsrccod2/A-Law Compressor  A=87.6  V=1
  Abs : Abs  SaturateOnIntegerOverflow=off
  Gain1 : Gain  Gain=127
  Integer to Bit Converter : simulink/Logic and Bit Operations/Integer to Bit Converter  nbits=7  signedInputValues=Unsigned  bitOrder=MSB first  outDtype=Inherit via internal rule
      settings: LibrarySourceBlock=|
      | commutil2/Integer to Bit
      | Converter
  Mux : Mux  Inputs=2
  Quantizer : Quantizer  QuantizationInterval=1
  Relay : Relay
  Saturation : Saturate  UpperLimit=1  LowerLimit=-1
  Out1 : Outport
  wires:
  Integer to Bit Converter/1 -> Mux/2
  Mux/1 -> Out1/1
  A-Law Compressor/1 -> Gain1/1
  Gain1/1 -> Quantizer/1
  Quantizer/1 -> Integer to Bit Converter/1
  Saturation/1 -> Abs/1
  Relay/1 -> Mux/1
  Abs/1 -> Relay/1, A-Law Compressor/1
  In1/1 -> Saturation/1

== system v3/sourse by PCM_Encode/Subsystem ==
  In1 : Inport
  PCM_decode1 : Subsystem
  To Multimedia File : dspvision/To Multimedia File  outputFilename=G:\zizim\Documents\作业\audio_output\PCM_Decode.wav  streamSelection=Audio only  videoCompressor=None (uncompressed)  audioCompressor=None (uncompressed)  imagePorts=Separate color signals  fileType=WAV  audioDatatype=Determine from input data type  fourcc=RGB  videoQuality=75  mj2000CompFactor=10
      settings: LibrarySourceBlock=audiosinks/To Multimedia File
  Zero-Order Hold : ZeroOrderHold  SampleTime=-1
  Out1 : Outport
  Out2 : Outport  Port=2
  wires:
  PCM_decode1/1(Out1) -> Out1/1, Zero-Order Hold/1
  In1/1 -> PCM_decode1/1(In1)
  Zero-Order Hold/1 -> Out2/1, To Multimedia File/1

== system v3/Subsystem1/HDB3/+-1循环 ==
  Enable : EnablePort
  Constant1 : Constant  Value=-1
  Memory : Memory  InitialCondition=1  InheritSampleTime=on
  Product : Product  RndMeth=Zero
  Out1 : Outport
  wires:
  Constant1/1 -> Product/1
  Memory/1 -> Product/2
  Product/1 -> Memory/1, Out1/1

== system v3/Subsystem1/HDB3/Subsystem3 ==
  In2 : Inport
  Enable : EnablePort
  Out1 : Outport
  wires:
  In2/1 -> Out1/1

== system v3/Subsystem1/HDB3/保持上一个1的极性 ==
  In1 : Inport
  Enable : EnablePort  StatesWhenEnabling=reset
  Out1 : Outport
  wires:
  In1/1 -> Out1/1

== system v3/Subsystem1/HDB3/有1就乘以-1 ==
  Enable : EnablePort
  Constant1 : Constant  Value=-1
  Memory : Memory  InitialCondition=-1  InheritSampleTime=on
  Product : Product  RndMeth=Zero
  Out1 : Outport
  wires:
  Constant1/1 -> Product/1
  Memory/1 -> Product/2
  Product/1 -> Memory/1, Out1/1

== system v3/Subsystem1/HDB3/有一个2，就输出 ==
  In1 : Inport
  Enable : EnablePort  StatesWhenEnabling=reset
  Out1 : Outport
  wires:
  In1/1 -> Out1/1

== system v3/Subsystem1/HDB3/有几个零输出几，超过4就清0 输入0000000 输出1230123 ==
  Enable : EnablePort  StatesWhenEnabling=reset
  Add : Sum
  Constant : Constant
  Constant1 : Constant  Value=0
  Switch3 : Switch  Criteria=u2 > Threshold  Threshold=3  SaturateOnIntegerOverflow=off  InputSameDT=off
  Unit Delay : UnitDelay  SampleTime=-1  HasFrameUpgradeWarning=on
  Out1 : Outport
  wires:
  Constant/1 -> Add/1
  Add/1 -> Unit Delay/1
  Unit Delay/1 -> Switch3/2, Switch3/3
  Constant1/1 -> Switch3/1
  Switch3/1 -> Add/2, Out1/1

== system v3/Subsystem1/HDB3 解码模块/Subsystem1 ==
  In1 : Inport
  Enable : EnablePort  StatesWhenEnabling=reset
  Out1 : Outport
  wires:
  In1/1 -> Out1/1

== system v3/Subsystem1/抽样判决模块/判决 ==
  In1 : Inport
  Constant12 : Constant
  Constant13 : Constant  Value=0
  Constant14 : Constant  Value=-1
  Constant15 : Constant  Value=0
  Gain5 : Gain  Gain=-1
  Sum4 : Sum  Inputs=|++
  开关电路6 : Switch  Criteria=u2 > Threshold  Threshold=0.5  SaturateOnIntegerOverflow=off  InputSameDT=off
  开关电路7 : Switch  Criteria=u2 > Threshold  Threshold=0.5  SaturateOnIntegerOverflow=off  InputSameDT=off
  Out1 : Outport
  wires:
  Sum4/1 -> Out1/1
  In1/1 -> Gain5/1, 开关电路6/2
  Constant14/1 -> 开关电路7/1
  Constant13/1 -> 开关电路6/3
  开关电路6/1 -> Sum4/1
  开关电路7/1 -> Sum4/2
  Constant15/1 -> 开关电路7/3
  Constant12/1 -> 开关电路6/1
  Gain5/1 -> 开关电路7/2

== system v3/Subsystem1/抽样判决模块/每隔抽样 ==
  In1 : Inport
  Trigger : TriggerPort  VariantControl=Variant
  Out1 : Outport
  wires:
  In1/1 -> Out1/1

== system v3/sourse by PCM_Decode1/Subsystem/PCM_encode_d ==
  In1 : Inport
  A-Law Compressor : commsrccod2/A-Law Compressor  A=87.6  V=1
  Abs : Abs  SaturateOnIntegerOverflow=off
  Gain1 : Gain  Gain=127
  Integer to Bit Converter : simulink/Logic and Bit Operations/Integer to Bit Converter  nbits=7  signedInputValues=Unsigned  bitOrder=MSB first  outDtype=Inherit via internal rule
      settings: LibrarySourceBlock=|
      | commutil2/Integer to Bit
      | Converter
  Mux : Mux  Inputs=2
  Quantizer : Quantizer  QuantizationInterval=1
  Relay : Relay
  Saturation : Saturate  UpperLimit=1  LowerLimit=-1
  Out1 : Outport
  wires:
  Integer to Bit Converter/1 -> Mux/2
  Mux/1 -> Out1/1
  A-Law Compressor/1 -> Gain1/1
  Gain1/1 -> Quantizer/1
  Quantizer/1 -> Integer to Bit Converter/1
  Saturation/1 -> Abs/1
  Relay/1 -> Mux/1
  Abs/1 -> Relay/1, A-Law Compressor/1
  In1/1 -> Saturation/1

== system v3/sourse by PCM_Decode2/Subsystem/PCM_encode_d ==
  In1 : Inport
  A-Law Compressor : commsrccod2/A-Law Compressor  A=87.6  V=1
  Abs : Abs  SaturateOnIntegerOverflow=off
  Gain1 : Gain  Gain=127
  Integer to Bit Converter : simulink/Logic and Bit Operations/Integer to Bit Converter  nbits=7  signedInputValues=Unsigned  bitOrder=MSB first  outDtype=Inherit via internal rule
      settings: LibrarySourceBlock=|
      | commutil2/Integer to Bit
      | Converter
  Mux : Mux  Inputs=2
  Quantizer : Quantizer  QuantizationInterval=1
  Relay : Relay
  Saturation : Saturate  UpperLimit=1  LowerLimit=-1
  Out1 : Outport
  wires:
  Integer to Bit Converter/1 -> Mux/2
  Mux/1 -> Out1/1
  A-Law Compressor/1 -> Gain1/1
  Gain1/1 -> Quantizer/1
  Quantizer/1 -> Integer to Bit Converter/1
  Saturation/1 -> Abs/1
  Relay/1 -> Mux/1
  Abs/1 -> Relay/1, A-Law Compressor/1
  In1/1 -> Saturation/1

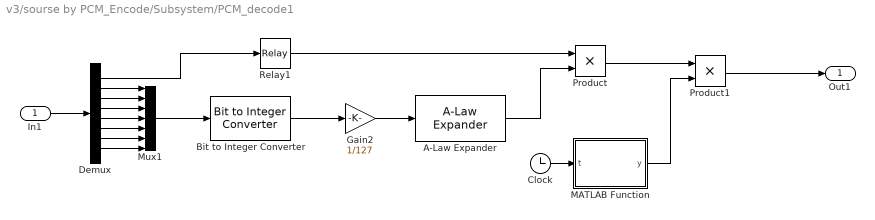
== system v3/sourse by PCM_Encode/Subsystem/PCM_decode1 ==
  In1 : Inport
  A-Law Expander : commsrccod2/A-Law Expander  A=87.6  V=1
  Bit to Integer Converter : simulink/Logic and Bit Operations/Bit to Integer Converter  nbits=7  bitOrder=MSB first  signedOutputValues=Unsigned  outDtype=double  outDtypeSigned=Inherit via internal rule
      settings: LibrarySourceBlock=|
      | commutil2/Bit to Integer
      | Converter
  Clock : Clock
      settings: Decimation=4
  Demux : Demux  Outputs=8
  Gain2 : Gain  Gain=1/127
  MATLAB Function : MATLAB Function  TreatAsAtomicUnit=on
  Mux1 : Mux  Inputs=7
  Product : Product
  Product1 : Product
  Relay1 : Relay  OnSwitchValue=0.9  OffOutputValue=-1
  Out1 : Outport
  wires:
  In1/1 -> Demux/1
  Relay1/1 -> Product/1
  Demux/5 -> Mux1/4
  Mux1/1 -> Bit to Integer Converter/1
  Demux/1 -> Relay1/1
  Demux/4 -> Mux1/3
  Gain2/1 -> A-Law Expander/1
  Demux/6 -> Mux1/5
  Demux/7 -> Mux1/6
  Bit to Integer Converter/1 -> Gain2/1
  Demux/2 -> Mux1/1
  Demux/3 -> Mux1/2
  A-Law Expander/1 -> Product/2
  Demux/8 -> Mux1/7
  Product/1 -> Product1/1
  Product1/1 -> Out1/1
  MATLAB Function/1(y) -> Product1/2
  Clock/1 -> MATLAB Function/1(t)

== matlab function v3/sourse by PCM_Encode/Subsystem/PCM_decode1/MATLAB Function ==
  data: t input; y output
function y = rect_wave(t)
    % 生成周期为1/(4*pi)、占空比50%、幅度在-1和1之间的矩形波
    % 输入t：Simulink仿真时间（需将模块输入连接到Clock模块的输出）
    
    T = 1/8000;  % 周期
    duty = 0.5;    % 占空比50%
    
    % 计算归一化时间（在0到周期内的位置）
    t_norm = mod(t, T);
    
    % 生成矩形波：前半周期为1，后半周期为-1
    if t_norm < duty * T
        y = 1;
    else
        y = -1;
    end
end

== matlab function v3/sourse by PCM_Decode1/PCM_decode1/MATLAB Function ==
  data: t input; y output
function y = rect_wave(t)
    % 生成周期为1/(4*pi)、占空比50%、幅度在-1和1之间的矩形波
    % 输入t：Simulink仿真时间（需将模块输入连接到Clock模块的输出）
    
    T = 1/8000;  % 周期
    duty = 0.5;    % 占空比50%
    
    % 计算归一化时间（在0到周期内的位置）
    t_norm = mod(t, T);
    
    % 生成矩形波：前半周期为1，后半周期为-1
    if t_norm < duty * T
        y = 1;
    else
        y = -1;
    end
end

== matlab function v3/sourse by PCM_Decode1/Subsystem/MATLAB Function ==
  data: t input; y output
function y = rect_wave(t)
    % 生成周期为1/(4*pi)、占空比50%、幅度在-1和1之间的矩形波
    % 输入t：Simulink仿真时间（需将模块输入连接到Clock模块的输出）
    
    T = 1/8000;  % 周期
    duty = 0.5;    % 占空比50%
    
    % 计算归一化时间（在0到周期内的位置）
    t_norm = mod(t, T);
    
    % 生成矩形波：前半周期为1，后半周期为-1
    if t_norm < duty * T
        y = 1;
    else
        y = -1;
    end
end

== matlab function v3/sourse by PCM_Encode/MATLAB Function ==
  data: t input; y output
function y = rect_wave(t)
    % 生成、占空比50%、幅度在-1和1之间的矩形波
    % 输入t：Simulink仿真时间（需将模块输入连接到Clock模块的输出）
    
    T = 1/8000;  % 周期
    duty = 0.5;    % 占空比50%
    
    % 计算归一化时间（在0到周期内的位置）
    t_norm = mod(t, T);
    
    % 生成矩形波：前半周期为1，后半周期为-1
    if t_norm < duty * T
        y = 1;
    else
        y = -1;
    end
end

== matlab function v3/sourse by PCM_Decode2/Subsystem/MATLAB Function ==
  data: t input; y output
function y = rect_wave(t)
    % 生成周期为1/(4*pi)、占空比50%、幅度在-1和1之间的矩形波
    % 输入t：Simulink仿真时间（需将模块输入连接到Clock模块的输出）
    
    T = 1/8000;  % 周期
    duty = 0.5;    % 占空比50%
    
    % 计算归一化时间（在0到周期内的位置）
    t_norm = mod(t, T);
    
    % 生成矩形波：前半周期为1，后半周期为-1
    if t_norm < duty * T
        y = 1;
    else
        y = -1;
    end
end

== matlab function v3/sourse by PCM_Decode2/PCM_decode1/MATLAB Function ==
  data: t input; y output
function y = rect_wave(t)
    % 生成周期为1/(4*pi)、占空比50%、幅度在-1和1之间的矩形波
    % 输入t：Simulink仿真时间（需将模块输入连接到Clock模块的输出）
    
    T = 1/8000;  % 周期
    duty = 0.5;    % 占空比50%
    
    % 计算归一化时间（在0到周期内的位置）
    t_norm = mod(t, T);
    
    % 生成矩形波：前半周期为1，后半周期为-1
    if t_norm < duty * T
        y = 1;
    else
        y = -1;
    end
end
